simulink model "audiomultibanddynamiccompression"  (R2021b)
settings: Solver=FixedStepDiscrete  StartTime=0.0  StopTime=Inf  RelTol=1e-3  EnableMultiTasking=on
InitFcn:
  | Ts = 1/44.1e3;
  | L = 4096;
values from neighbouring files (symbols this model uses):
  audio = HelperMultibandCompressionSim(S)    [DynamicEQ_Prototype_OUT.m]    (also in HelperMultibandCompressionSim.m = SC)
libraries: dspindex x8, audiodynamicrange x4, dspstat3 x2, dspsnks4 x1, audiofilters x1, dspvision x1
CloseFcn:
  | clear Ts L
  | close all force
settings Model: Creator=The MathWorks, Inc.  LastModifiedBy=nikid
settings SolverCC: AlgebraicLoopSolver=TrustRegion
settings DataIOCC: LimitDataPoints=on  SaveFormat=Array  ReturnWorkspaceOutputs=off
settings OptimizationCC: LifeSpan=inf
settings DebuggingCC: UnderspecifiedInitializationDetection=Classic  MergeDetectMultiDrivingBlocksExec=none  SolverPrmCheckMsg=warning  AllowSymbolicDim=off  SFUnexpectedBacktrackingDiag=warning  SFNoUnconditionalDefaultTransitionDiag=warning  SFExecutionAtInitializationDiag=none  SFMachineParentedDataDiag=warning  ArithmeticOperatorsInVariantConditions=warning
settings HardwareCC: ProdBitPerPointer=32  ProdBitPerSizeT=32  ProdBitPerPtrDiffT=32  ProdLargestAtomicFloat=None  ProdIntDivRoundTo=Undefined  ProdEndianess=Unspecified  ProdWordSize=32  ProdHWDeviceType=32-bit Generic
settings ModelReferenceCC: PropagateSignalLabelsOutOfModel=off
settings SFSimCC: SimUseLocalCustomCode=off  CustomCodeUndefinedFunction=UseInterfaceOnly
settings RTWCC: RTWUseLocalCustomCode=off
settings CodeAppCC: StateflowObjectComments=on
settings GRTTargetCC: TargetLangStandard=C89/C90 (ANSI)
settings ConfigComp: CovMetricSettings=dw  CovSaveCumulativeToWorkspaceVar=on  CovSaveSingleToWorkspaceVar=on  CovExternalEMLEnable=off  CovSFcnEnable=off

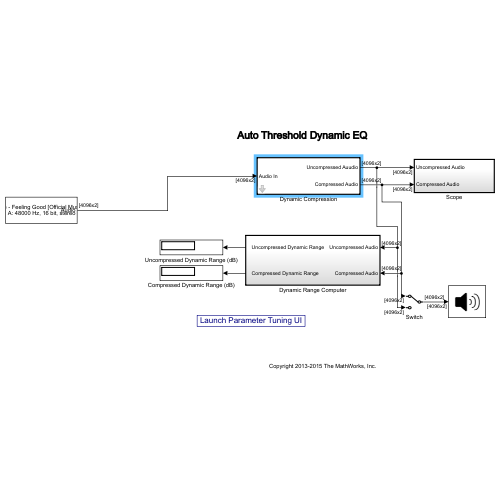
[thumbnail: Simulink's stored preview of the top-level diagram]
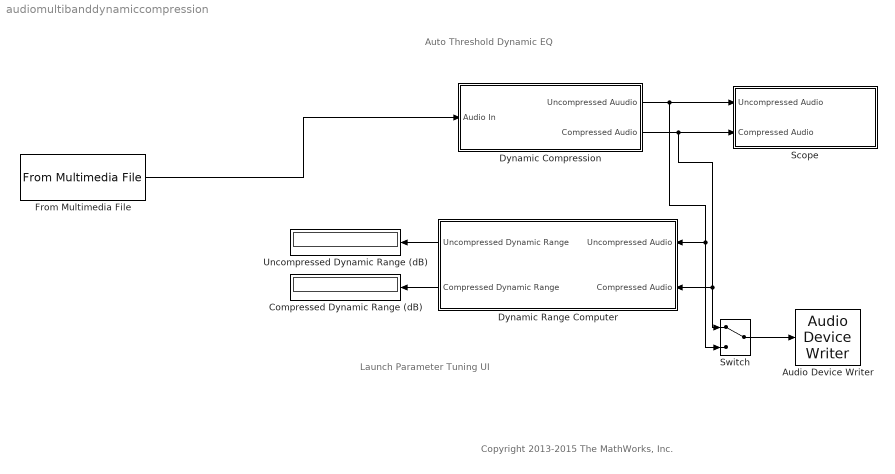
== system audiomultibanddynamiccompression ==
  note: Copyright 2013-2015 The MathWorks, Inc.
  note: Launch Parameter Tuning UI
  note: Auto Threshold Dynamic EQ
  Audio Device Writer : dspsnks4/Audio Device Writer  Driver=DirectSound  Device=Default  InheritSampleRate=on  SampleRate=44100  BitDepth=16-bit integer  BufferSize=4096  NumBuffers=10  DefaultOutputChannelMapping=on  OutputChannelMapping=1:2  OutputNumUnderrunSamples=off  DriverIdx=1  DeviceWarnFlag=''
  Compressed Dynamic Range (dB) : Display
  Dynamic Compression : Subsystem  TreatAsAtomicUnit=on  mask(Multiband Compressor){T1=-5, CF1=5.0, TA1=0.005, TR1=0.1, T2=-10.0, CF2=5.0, TA2=0.005, TR2=0.1, T3=-20, CF3=5.0, TA3=0.002, TR3=0.050, T4=-30, CF4=4, TA4=0.002, TR4=0.050}
      mask prompts: T1 "audio:dynamicrange:Threshold_MP"; CF1 "audio:dynamicrange:Ratio_MP"; TA1 "audio:dynamicrange:AttackTime_MP"; TR1 "audio:dynamicrange:ReleaseTime_MP"; T2 "audio:dynamicrange:Threshold_MP"; CF2 "audio:dynamicrange:Ratio_MP"; TA2 "audio:dynamicrange:AttackTime_MP"; TR2 "audio:dynamicrange:ReleaseTime_MP"; T3 "audio:dynamicrange:Threshold_MP"; CF3 "audio:dynamicrange:Ratio_MP"; TA3 "audio:dynamicrange:AttackTime_MP"; TR3 "audio:dynamicrange:ReleaseTime_MP"; T4 "audio:dynamicrange:Threshold_MP"; CF4 "audio:dynamicrange:Ratio_MP"; TA4 "audio:dynamicrange:AttackTime_MP"; TR4 "audio:dynamicrange:ReleaseTime_MP"
      mask help: Multiband Compressor
      mask TypeOptions T1: Compressor Bank/Compressor1/Threshold
      mask TypeOptions CF1: Compressor Bank/Compressor1/Ratio
      mask TypeOptions TA1: Compressor Bank/Compressor1/AttackTime
      mask TypeOptions TR1: Compressor Bank/Compressor1/ReleaseTime
      mask TypeOptions T2: Compressor Bank/Compressor2/Threshold
      mask TypeOptions CF2: Compressor Bank/Compressor2/Ratio
      mask TypeOptions TA2: Compressor Bank/Compressor2/AttackTime
      mask TypeOptions TR2: Compressor Bank/Compressor2/ReleaseTime
      mask TypeOptions T3: Compressor Bank/Compressor3/Threshold
      mask TypeOptions CF3: Compressor Bank/Compressor3/Ratio
      mask TypeOptions TA3: Compressor Bank/Compressor3/AttackTime
      mask TypeOptions TR3: Compressor Bank/Compressor3/ReleaseTime
      mask TypeOptions T4: Compressor Bank/Compressor4/Threshold
      mask TypeOptions CF4: Compressor Bank/Compressor4/Ratio
      mask TypeOptions TA4: Compressor Bank/Compressor4/AttackTime
      mask TypeOptions TR4: Compressor Bank/Compressor4/ReleaseTime
      mask DialogControl Container3 Prompt: Band 1
      mask DialogControl T1 Prompt: Threshold (dB):
      mask DialogControl CF1 Prompt: Ratio:
      mask DialogControl TA1 Prompt: Attack time (s):
      mask DialogControl TR1 Prompt: Release time (s):
      mask DialogControl Container5 Prompt: Band 2
      mask DialogControl T2 Prompt: Threshold (dB):
      mask DialogControl CF2 Prompt: Ratio:
      mask DialogControl TA2 Prompt: Attack time (s):
      mask DialogControl TR2 Prompt: Release time (s):
      mask DialogControl Container8 Prompt: Band 3
      mask DialogControl T3 Prompt: Threshold (dB):
      mask DialogControl CF3 Prompt: Ratio:
      mask DialogControl TA3 Prompt: Attack time (s):
      mask DialogControl TR3 Prompt: Release time (s):
      mask DialogControl Container9 Prompt: Band 4
      mask DialogControl T4 Prompt: Threshold (dB):
      mask DialogControl CF4 Prompt: Ratio:
      mask DialogControl TA4 Prompt: Attack time (s):
      mask DialogControl TR4 Prompt: Release time (s):
  Dynamic Range Computer : Subsystem  TreatAsAtomicUnit=on
  From Multimedia File : dspvision/From Multimedia File  inputFilename=D:\OneDrive - Politecnico di Torino\Università D\Materiale D\Tesi\Tesi Git\DynamicEQ_Tesi\Sample audio\Michael Bublé - Feeling Good [Official Music Video].wav  readRange=[1 Inf]  loop=on  numPlays=inf  outputStreams=Audio only  videoDataType=single  audioDataType=double  inheritSampleTime=on  userDefinedSampleTime=1/30  noAudioOutput=off  isIntensityVideo=off  fourcc=RGB  colorVideoFormat=Separate color signals  outputEOF=off  dataOrg=Column-major  audioFrameSize=L  computeAudioFrameSize=off  outSamplingMode=Sample based
  Scope : Subsystem  TreatAsAtomicUnit=on
  Switch : ManualSwitch
  Uncompressed Dynamic Range (dB) : Display
  wires:
  From Multimedia File/1 -> Dynamic Compression/1(Audio In)
  Dynamic Compression/1("  Uncompressed Auudio") -> Switch/2, Dynamic Range Computer/1(Uncompressed Audio), Scope/1(Uncompressed Audio)
  Dynamic Compression/2("   Compressed Audio") -> Switch/1, Dynamic Range Computer/2(Compressed Audio), Scope/2(Compressed Audio)
  Switch/1 -> Audio Device Writer/1
  Dynamic Range Computer/1("   Uncompressed Dynamic Range") -> Uncompressed Dynamic Range (dB)/1
  Dynamic Range Computer/2("   Compressed Dynamic Range") -> Compressed Dynamic Range (dB)/1

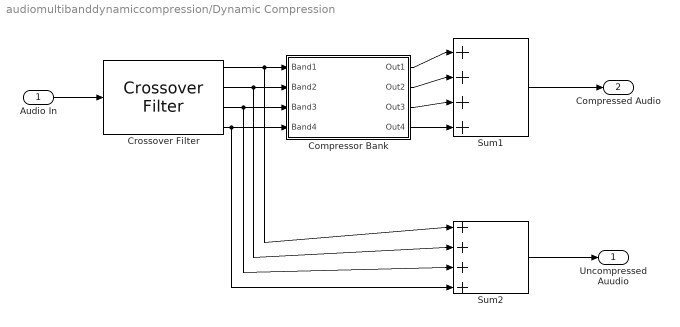
== system audiomultibanddynamiccompression/Dynamic Compression ==
  Audio In : Inport
  Compressor Bank : Subsystem  TreatAsAtomicUnit=on
  Crossover Filter : audiofilters/Crossover Filter  NCrossovers=3  Crossover1Port=off  Crossover1=100  Order1Port=off  Order1=2  Crossover2Port=off  Crossover2=800  Order2Port=off  Order2=2  Crossover3Port=off  Crossover3=1500  Order3Port=off  Order3=2  Crossover4Port=off  Crossover4=3000  Order4Port=off  Order4=2  InheritSampleRate=off  SampleRate=44100  SimulateUsing=Interpreted execution
      settings: SourceProductBaseCode=AU
  Sum1 : Sum  Inputs=|++++
  Sum2 : Sum  Inputs=|++++
  "  Uncompressed Auudio" : Outport  VectorParamsAs1DForOutWhenUnconnected=off
  "   Compressed Audio" : Outport  Port=2  VectorParamsAs1DForOutWhenUnconnected=off
  wires:
  Audio In/1 -> Crossover Filter/1
  Sum2/1 -> "  Uncompressed Auudio"/1
  Sum1/1 -> "   Compressed Audio"/1
  Compressor Bank/1(Out1) -> Sum1/1
  Compressor Bank/2(Out2) -> Sum1/2
  Compressor Bank/3(Out3) -> Sum1/3
  Compressor Bank/4(Out4) -> Sum1/4
  Crossover Filter/3 -> Sum2/3, Compressor Bank/3(Band3)
  Crossover Filter/2 -> Sum2/2, Compressor Bank/2(Band2)
  Crossover Filter/1 -> Sum2/1, Compressor Bank/1(Band1)
  Crossover Filter/4 -> Sum2/4, Compressor Bank/4(Band4)

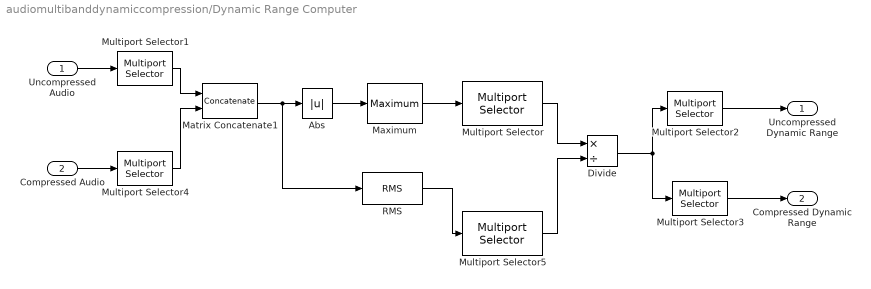
== system audiomultibanddynamiccompression/Dynamic Range Computer ==
  Uncompressed Audio : Inport
  Compressed Audio : Inport  Port=2
  Abs : Abs
  Divide : Product  Inputs=*/
  Matrix Concatenate1 : Concatenate  Mode=Multidimensional array  ConcatenateDimension=2
  Maximum : dspstat3/Maximum  operation=maximum  fcn=Running  indexBase=One  operateOver=Each column  Dimension=1  InputProcessing=Columns as channels (frame based)  reset=None  roiEnable=off  roiType=Rectangles  roiPortion=Entire ROI  roiOutput=Individual statistics for each ROI  roiFlag=off  roundingMode=Floor  overflowMode=off  accumDataTypeStr=Inherit: Same as product output  accumLastDataTypeStr=Inherit: Same as product output
  Multiport Selector : dspindex/Multiport Selector  rowsOrCols=Rows  idxCellArray={L}  idxErrMode=Clip Index
  Multiport Selector1 : dspindex/Multiport Selector  rowsOrCols=Columns  idxCellArray={1}  idxErrMode=Clip Index
  Multiport Selector2 : dspindex/Multiport Selector  rowsOrCols=Columns  idxCellArray={1}  idxErrMode=Clip Index
  Multiport Selector3 : dspindex/Multiport Selector  rowsOrCols=Columns  idxCellArray={2}  idxErrMode=Clip Index
  Multiport Selector4 : dspindex/Multiport Selector  rowsOrCols=Columns  idxCellArray={1}  idxErrMode=Clip Index
  Multiport Selector5 : dspindex/Multiport Selector  rowsOrCols=Rows  idxCellArray={L}  idxErrMode=Clip Index
  RMS : dspstat3/RMS  run=on  directionMode=Each column  dimension=1  InputProcessing=Columns as channels (frame based)  reset_popup=None
  "   Uncompressed Dynamic Range" : Outport  VectorParamsAs1DForOutWhenUnconnected=off
  "   Compressed Dynamic Range" : Outport  Port=2  VectorParamsAs1DForOutWhenUnconnected=off
  wires:
  Uncompressed Audio/1 -> Multiport Selector1/1
  Compressed Audio/1 -> Multiport Selector4/1
  Multiport Selector1/1 -> Matrix Concatenate1/1
  Multiport Selector4/1 -> Matrix Concatenate1/2
  Matrix Concatenate1/1 -> RMS/1, Abs/1
  Multiport Selector2/1 -> "   Uncompressed Dynamic Range"/1
  Multiport Selector3/1 -> "   Compressed Dynamic Range"/1
  Abs/1 -> Maximum/1
  Maximum/1 -> Multiport Selector/1
  RMS/1 -> Multiport Selector5/1
  Multiport Selector/1 -> Divide/1
  Multiport Selector5/1 -> Divide/2
  Divide/1 -> Multiport Selector2/1, Multiport Selector3/1

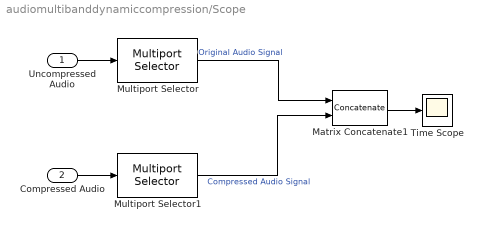
== system audiomultibanddynamiccompression/Scope ==
  Uncompressed Audio : Inport
  Compressed Audio : Inport  Port=2
  Matrix Concatenate1 : Concatenate  Mode=Multidimensional array  ConcatenateDimension=2
  Multiport Selector : dspindex/Multiport Selector  rowsOrCols=Columns  idxCellArray={ 1 }  idxErrMode=Clip Index
  Multiport Selector1 : dspindex/Multiport Selector  rowsOrCols=Columns  idxCellArray={ 1 }  idxErrMode=Clip Index
  Time Scope : Scope
  wires:
  Multiport Selector/1 -> Matrix Concatenate1/1  "Original Audio Signal"
  Multiport Selector1/1 -> Matrix Concatenate1/2  "Compressed Audio Signal"
  Matrix Concatenate1/1 -> Time Scope/1
  Compressed Audio/1 -> Multiport Selector1/1
  Uncompressed Audio/1 -> Multiport Selector/1

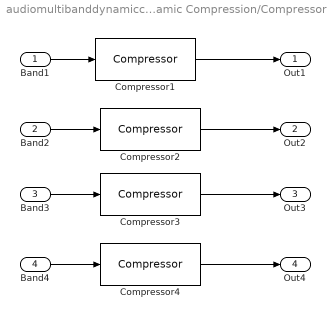
== system audiomultibanddynamiccompression/Dynamic Compression/Compressor Bank ==
  Band1 : Inport
  Band2 : Inport  Port=2
  Band3 : Inport  Port=3
  Band4 : Inport  Port=4
  Compressor1 : audiodynamicrange/Compressor  ThresholdPort=off  Threshold=-5  RatioPort=off  Ratio=5.0  KneeWidthPort=off  KneeWidth=0.0  AttackTimePort=off  AttackTime=0.005  ReleaseTimePort=off  ReleaseTime=0.1  MakeUpGainMode=Property  MakeUpGain=0.0  InheritSampleRate=off  SampleRate=44100  outputGain=off  EnableSidechain=off  SimulateUsing=Interpreted execution
      settings: SourceProductBaseCode=AU
  Compressor2 : audiodynamicrange/Compressor  ThresholdPort=off  Threshold=-10.0  RatioPort=off  Ratio=5.0  KneeWidthPort=off  KneeWidth=0.0  AttackTimePort=off  AttackTime=0.005  ReleaseTimePort=off  ReleaseTime=0.1  MakeUpGainMode=Property  MakeUpGain=0.0  InheritSampleRate=off  SampleRate=44100  outputGain=off  EnableSidechain=off  SimulateUsing=Interpreted execution
      settings: SourceProductBaseCode=AU
  Compressor3 : audiodynamicrange/Compressor  ThresholdPort=off  Threshold=-20  RatioPort=off  Ratio=5.0  KneeWidthPort=off  KneeWidth=0.0  AttackTimePort=off  AttackTime=0.002  ReleaseTimePort=off  ReleaseTime=0.050  MakeUpGainMode=Property  MakeUpGain=0.0  InheritSampleRate=off  SampleRate=44100  outputGain=off  EnableSidechain=off  SimulateUsing=Interpreted execution
      settings: SourceProductBaseCode=AU
  Compressor4 : audiodynamicrange/Compressor  ThresholdPort=off  Threshold=-30  RatioPort=off  Ratio=4  KneeWidthPort=off  KneeWidth=0.0  AttackTimePort=off  AttackTime=0.002  ReleaseTimePort=off  ReleaseTime=0.050  MakeUpGainMode=Property  MakeUpGain=0.0  InheritSampleRate=off  SampleRate=44100  outputGain=off  EnableSidechain=off  SimulateUsing=Interpreted execution
      settings: SourceProductBaseCode=AU
  Out1 : Outport  VectorParamsAs1DForOutWhenUnconnected=off
  Out2 : Outport  Port=2  VectorParamsAs1DForOutWhenUnconnected=off
  Out3 : Outport  Port=3  VectorParamsAs1DForOutWhenUnconnected=off
  Out4 : Outport  Port=4  VectorParamsAs1DForOutWhenUnconnected=off
  wires:
  Band1/1 -> Compressor1/1
  Band2/1 -> Compressor2/1
  Band3/1 -> Compressor3/1
  Band4/1 -> Compressor4/1
  Compressor1/1 -> Out1/1
  Compressor2/1 -> Out2/1
  Compressor3/1 -> Out3/1
  Compressor4/1 -> Out4/1
